simulink model "db6_4_Level_double"  (R2021a)
settings: Solver=VariableStepAuto  StartTime=0.0  StopTime=8  RelTol=1e-3
undefined symbols (not defined in the file): lambda2
libraries: dspsigops x9, dspquant2 x1
(part 2 of 3)

== system db6_4_Level_double/2nd_Level_Decomp/LoD_Even ==
  In_LoD_e : Inport  OutDataTypeStr=double  SampleTime=1/44100
  Add{,1..4} (5 alike) : Sum  AccumDataTypeStr=double  OutDataTypeStr=double
  Delay{,1..9} (10 alike) : Delay  DelayLength=1  SampleTime=1/44100
  LoD_0 : Constant  Value=-0.001077301  OutDataTypeStr=double  SampleTime=1/44100
  LoD_10 : Constant  Value=0.49462389  OutDataTypeStr=double  SampleTime=1/44100
  LoD_2 : Constant  Value=0.000553842  OutDataTypeStr=double  SampleTime=1/44100
  LoD_4 : Constant  Value=0.027522866  OutDataTypeStr=double  SampleTime=1/44100
  LoD_6 : Constant  Value=-0.129766868  OutDataTypeStr=double  SampleTime=1/44100
  LoD_8 : Constant  Value=0.315250352  OutDataTypeStr=double  SampleTime=1/44100
  Multiply{,1..5} (6 alike) : Product  OutDataTypeStr=double
  Rate Transition{,1..4} (5 alike) : RateTransition  OutPortSampleTime=1/44100
  Out_LoD_e : Outport  OutDataTypeStr=double  SampleTime=1/44100  VectorParamsAs1DForOutWhenUnconnected=off
  wires:
  Multiply3/1 -> Add3/1
  Add/1 -> Out_LoD_e/1
  Rate Transition3/1 -> Delay8/1, Multiply4/2
  Add3/1 -> Delay4/1
  In_LoD_e/1 -> Delay/1, Multiply/2
  Multiply2/1 -> Add2/1
  Multiply/1 -> Add/1
  Rate Transition1/1 -> Delay5/1, Multiply2/2
  Delay/1 -> Rate Transition/1
  Delay2/1 -> Add1/2
  Delay3/1 -> Add/2
  Delay7/1 -> Add3/2
  Add2/1 -> Delay2/1
  Add1/1 -> Delay3/1
  Rate Transition2/1 -> Delay6/1, Multiply3/2
  Delay1/1 -> Rate Transition1/1
  LoD_10/1 -> Multiply5/1
  Rate Transition/1 -> Delay1/1, Multiply1/2
  LoD_4/1 -> Multiply2/1
  Delay5/1 -> Rate Transition2/1
  LoD_0/1 -> Multiply/1
  LoD_2/1 -> Multiply1/1
  Delay8/1 -> Rate Transition4/1
  Rate Transition4/1 -> Multiply5/2
  Multiply4/1 -> Add4/1
  Delay4/1 -> Add2/2
  Delay9/1 -> Add4/2
  Multiply5/1 -> Delay9/1
  Delay6/1 -> Rate Transition3/1
  Add4/1 -> Delay7/1
  LoD_8/1 -> Multiply4/1
  LoD_6/1 -> Multiply3/1
  Multiply1/1 -> Add1/1

== system db6_4_Level_double/2nd_Level_Decomp/LoD_Odd ==
  In_LoD_o : Inport  OutDataTypeStr=double  SampleTime=1/44100
  Add{,1..4} (5 alike) : Sum  AccumDataTypeStr=double  OutDataTypeStr=double
  Delay{,1..9} (10 alike) : Delay  DelayLength=1  SampleTime=1/44100
  LoD_1 : Constant  Value=0.004777258  OutDataTypeStr=double  SampleTime=1/44100
  LoD_11 : Constant  Value=0.111540743  OutDataTypeStr=double  SampleTime=1/44100
  LoD_3 : Constant  Value=-0.031582039  OutDataTypeStr=double  SampleTime=1/44100
  LoD_5 : Constant  Value=0.097501606  OutDataTypeStr=double  SampleTime=1/44100
  LoD_7 : Constant  Value=-0.226264694  OutDataTypeStr=double  SampleTime=1/44100
  LoD_9 : Constant  Value=0.751133908  OutDataTypeStr=double  SampleTime=1/44100
  Multiply{,1..5} (6 alike) : Product  OutDataTypeStr=double
  Rate Transition{,1..4} (5 alike) : RateTransition  OutPortSampleTime=1/44100
  Out_LoD_o : Outport  OutDataTypeStr=double  SampleTime=1/44100  VectorParamsAs1DForOutWhenUnconnected=off
  wires:
  LoD_1/1 -> Multiply/1
  Delay/1 -> Rate Transition/1
  Multiply4/1 -> Add4/1
  Delay2/1 -> Add1/2
  Rate Transition2/1 -> Delay6/1, Multiply3/2
  LoD_7/1 -> Multiply3/1
  Delay7/1 -> Add3/2
  Add2/1 -> Delay2/1
  Add1/1 -> Delay3/1
  Delay3/1 -> Add/2
  Multiply5/1 -> Delay9/1
  Rate Transition4/1 -> Multiply5/2
  Delay8/1 -> Rate Transition4/1
  Delay9/1 -> Add4/2
  Delay5/1 -> Rate Transition2/1
  Add4/1 -> Delay7/1
  Rate Transition3/1 -> Delay8/1, Multiply4/2
  LoD_9/1 -> Multiply4/1
  LoD_5/1 -> Multiply2/1
  Rate Transition/1 -> Delay1/1, Multiply1/2
  LoD_3/1 -> Multiply1/1
  Multiply3/1 -> Add3/1
  Delay1/1 -> Rate Transition1/1
  Add3/1 -> Delay4/1
  Multiply/1 -> Add/1
  Multiply1/1 -> Add1/1
  In_LoD_o/1 -> Delay/1, Multiply/2
  Delay6/1 -> Rate Transition3/1
  Delay4/1 -> Add2/2
  Add/1 -> Out_LoD_o/1
  LoD_11/1 -> Multiply5/1
  Multiply2/1 -> Add2/1
  Rate Transition1/1 -> Delay5/1, Multiply2/2

== system db6_4_Level_double/2nd_Level_Recon/HiR_Even ==
  In_HiR_e : Inport  OutDataTypeStr=double  SampleTime=1/44100
  Add{,1..4} (5 alike) : Sum  AccumDataTypeStr=double  OutDataTypeStr=double
  Delay{,1..9} (10 alike) : Delay  DelayLength=1  SampleTime=1/44100
  HiR_0 : Constant  Value=-0.001077301  OutDataTypeStr=double  SampleTime=1/44100
  HiR_10 : Constant  Value=0.49462389  OutDataTypeStr=double  SampleTime=1/44100
  HiR_2 : Constant  Value=0.000553842  OutDataTypeStr=double  SampleTime=1/44100
  HiR_4 : Constant  Value=0.027522866  OutDataTypeStr=double  SampleTime=1/44100
  HiR_6 : Constant  Value=-0.129766868  OutDataTypeStr=double  SampleTime=1/44100
  HiR_8 : Constant  Value=0.315250352  OutDataTypeStr=double  SampleTime=1/44100
  Multiply{,1..5} (6 alike) : Product  OutDataTypeStr=double
  Rate Transition{,1..4} (5 alike) : RateTransition  OutPortSampleTime=1/44100
  Out_HiR_e : Outport  OutDataTypeStr=double  SampleTime=1/44100  VectorParamsAs1DForOutWhenUnconnected=off
  wires:
  Delay3/1 -> Add/2
  In_HiR_e/1 -> Delay/1, Multiply/2
  HiR_4/1 -> Multiply2/1
  Multiply/1 -> Add/1
  Add1/1 -> Delay3/1
  Multiply1/1 -> Add1/1
  Delay2/1 -> Add1/2
  Add/1 -> Out_HiR_e/1
  HiR_0/1 -> Multiply/1
  HiR_2/1 -> Multiply1/1
  Delay1/1 -> Rate Transition1/1
  Rate Transition/1 -> Delay1/1, Multiply1/2
  Rate Transition1/1 -> Delay4/1, Multiply2/2
  Delay/1 -> Rate Transition/1
  Delay4/1 -> Rate Transition2/1
  HiR_6/1 -> Multiply3/1
  Multiply2/1 -> Add2/1
  Add2/1 -> Delay2/1
  Delay5/1 -> Add2/2
  HiR_8/1 -> Multiply4/1
  Rate Transition2/1 -> Delay6/1, Multiply3/2
  Delay6/1 -> Rate Transition3/1
  Add3/1 -> Delay5/1
  Multiply3/1 -> Add3/1
  Delay7/1 -> Add3/2
  HiR_10/1 -> Multiply5/1
  Rate Transition3/1 -> Delay8/1, Multiply4/2
  Rate Transition4/1 -> Multiply5/2
  Delay8/1 -> Rate Transition4/1
  Multiply5/1 -> Delay9/1
  Add4/1 -> Delay7/1
  Multiply4/1 -> Add4/1
  Delay9/1 -> Add4/2

== system db6_4_Level_double/2nd_Level_Recon/HiR_Odd ==
  In_HiR_o : Inport  OutDataTypeStr=double  SampleTime=1/44100
  Add{,1..4} (5 alike) : Sum  AccumDataTypeStr=double  OutDataTypeStr=double
  Delay{,1..9} (10 alike) : Delay  DelayLength=1  SampleTime=1/44100
  HiR_1 : Constant  Value=-0.004777258  OutDataTypeStr=double  SampleTime=1/44100
  HiR_11 : Constant  Value=-0.111540743  OutDataTypeStr=double  SampleTime=1/44100
  HiR_3 : Constant  Value=0.031582039  OutDataTypeStr=double  SampleTime=1/44100
  HiR_5 : Constant  Value=-0.097501606  OutDataTypeStr=double  SampleTime=1/44100
  HiR_7 : Constant  Value=0.226264694  OutDataTypeStr=double  SampleTime=1/44100
  HiR_9 : Constant  Value=-0.751133908  OutDataTypeStr=double  SampleTime=1/44100
  Multiply{,1..5} (6 alike) : Product  OutDataTypeStr=double
  Rate Transition{,1..4} (5 alike) : RateTransition  OutPortSampleTime=1/44100
  Out_HiR_o : Outport  OutDataTypeStr=double  SampleTime=1/44100  VectorParamsAs1DForOutWhenUnconnected=off
  wires:
  HiR_7/1 -> Multiply3/1
  HiR_3/1 -> Multiply1/1
  Delay2/1 -> Add1/2
  Delay/1 -> Rate Transition/1
  Delay5/1 -> Add2/2
  HiR_5/1 -> Multiply2/1
  Delay4/1 -> Rate Transition2/1
  Delay3/1 -> Add/2
  Add2/1 -> Delay2/1
  Multiply/1 -> Add/1
  Multiply1/1 -> Add1/1
  Rate Transition2/1 -> Delay6/1, Multiply3/2
  HiR_1/1 -> Multiply/1
  Multiply5/1 -> Delay9/1
  Delay1/1 -> Rate Transition1/1
  Delay8/1 -> Rate Transition4/1
  Add1/1 -> Delay3/1
  Add4/1 -> Delay7/1
  Delay9/1 -> Add4/2
  Rate Transition1/1 -> Delay4/1, Multiply2/2
  Add3/1 -> Delay5/1
  Delay6/1 -> Rate Transition3/1
  Rate Transition/1 -> Delay1/1, Multiply1/2
  HiR_9/1 -> Multiply4/1
  Multiply4/1 -> Add4/1
  Delay7/1 -> Add3/2
  Multiply3/1 -> Add3/1
  Multiply2/1 -> Add2/1
  HiR_11/1 -> Multiply5/1
  Rate Transition3/1 -> Delay8/1, Multiply4/2
  Add/1 -> Out_HiR_o/1
  In_HiR_o/1 -> Delay/1, Multiply/2
  Rate Transition4/1 -> Multiply5/2

== system db6_4_Level_double/2nd_Level_Recon/LoR_Even ==
  In_LoR_e : Inport  OutDataTypeStr=double  SampleTime=1/44100
  Add{,1..4} (5 alike) : Sum  AccumDataTypeStr=double  OutDataTypeStr=double
  Delay{,1..9} (10 alike) : Delay  DelayLength=1  SampleTime=1/44100
  LoR_0 : Constant  Value=0.111540743  OutDataTypeStr=double  SampleTime=1/44100
  LoR_10 : Constant  Value=0.004777258  OutDataTypeStr=double  SampleTime=1/44100
  LoR_2 : Constant  Value=0.751133908  OutDataTypeStr=double  SampleTime=1/44100
  LoR_4 : Constant  Value=-0.226264694  OutDataTypeStr=double  SampleTime=1/44100
  LoR_6 : Constant  Value=0.097501606  OutDataTypeStr=double  SampleTime=1/44100
  LoR_8 : Constant  Value=-0.031582039  OutDataTypeStr=double  SampleTime=1/44100
  Multiply{,1..5} (6 alike) : Product  OutDataTypeStr=double
  Rate Transition{,1..4} (5 alike) : RateTransition  OutPortSampleTime=1/44100
  Out_LoR_e : Outport  OutDataTypeStr=double  SampleTime=1/44100  VectorParamsAs1DForOutWhenUnconnected=off
  wires:
  Multiply5/1 -> Delay9/1
  LoR_6/1 -> Multiply3/1
  Rate Transition2/1 -> Delay6/1, Multiply3/2
  Multiply1/1 -> Add1/1
  Multiply/1 -> Add/1
  LoR_8/1 -> Multiply4/1
  Rate Transition3/1 -> Delay8/1, Multiply4/2
  Add2/1 -> Delay2/1
  Delay5/1 -> Add2/2
  Multiply2/1 -> Add2/1
  Delay3/1 -> Add/2
  Delay4/1 -> Rate Transition2/1
  Delay2/1 -> Add1/2
  Delay/1 -> Rate Transition/1
  In_LoR_e/1 -> Delay/1, Multiply/2
  Rate Transition/1 -> Delay1/1, Multiply1/2
  Add1/1 -> Delay3/1
  Add3/1 -> Delay5/1
  Delay8/1 -> Rate Transition4/1
  Delay1/1 -> Rate Transition1/1
  Delay6/1 -> Rate Transition3/1
  Rate Transition1/1 -> Delay4/1, Multiply2/2
  Delay9/1 -> Add4/2
  LoR_4/1 -> Multiply2/1
  Add4/1 -> Delay7/1
  LoR_0/1 -> Multiply/1
  Rate Transition4/1 -> Multiply5/2
  Multiply3/1 -> Add3/1
  Multiply4/1 -> Add4/1
  LoR_2/1 -> Multiply1/1
  Delay7/1 -> Add3/2
  LoR_10/1 -> Multiply5/1
  Add/1 -> Out_LoR_e/1

== system db6_4_Level_double/2nd_Level_Recon/LoR_Odd ==
  In_LoR_o : Inport  OutDataTypeStr=double  SampleTime=1/44100
  Add{,1..4} (5 alike) : Sum  AccumDataTypeStr=double  OutDataTypeStr=double
  Delay{,1..9} (10 alike) : Delay  DelayLength=1  SampleTime=1/44100
  LoR_1 : Constant  Value=0.49462389  OutDataTypeStr=double  SampleTime=1/44100
  LoR_11 : Constant  Value=-0.001077301  OutDataTypeStr=double  SampleTime=1/44100
  LoR_3 : Constant  Value=0.315250352  OutDataTypeStr=double  SampleTime=1/44100
  LoR_5 : Constant  Value=-0.129766868  OutDataTypeStr=double  SampleTime=1/44100
  LoR_7 : Constant  Value=0.027522866  OutDataTypeStr=double  SampleTime=1/44100
  LoR_9 : Constant  Value=0.000553842  OutDataTypeStr=double  SampleTime=1/44100
  Multiply{,1..5} (6 alike) : Product  OutDataTypeStr=double
  Rate Transition{,1..4} (5 alike) : RateTransition  OutPortSampleTime=1/44100
  Out_LoR_o : Outport  OutDataTypeStr=double  SampleTime=1/44100  VectorParamsAs1DForOutWhenUnconnected=off
  wires:
  Rate Transition2/1 -> Delay6/1, Multiply3/2
  Delay3/1 -> Add/2
  Add2/1 -> Delay2/1
  Delay4/1 -> Rate Transition2/1
  Delay/1 -> Rate Transition/1
  Delay5/1 -> Add2/2
  Delay2/1 -> Add1/2
  LoR_5/1 -> Multiply2/1
  LoR_7/1 -> Multiply3/1
  LoR_1/1 -> Multiply/1
  Multiply5/1 -> Delay9/1
  Multiply4/1 -> Add4/1
  LoR_11/1 -> Multiply5/1
  Rate Transition/1 -> Delay1/1, Multiply1/2
  Multiply/1 -> Add/1
  Delay6/1 -> Rate Transition3/1
  Add3/1 -> Delay5/1
  Rate Transition1/1 -> Delay4/1, Multiply2/2
  Add4/1 -> Delay7/1
  Delay9/1 -> Add4/2
  Add1/1 -> Delay3/1
  Delay8/1 -> Rate Transition4/1
  In_LoR_o/1 -> Delay/1, Multiply/2
  Add/1 -> Out_LoR_o/1
  Rate Transition3/1 -> Delay8/1, Multiply4/2
  Multiply1/1 -> Add1/1
  Rate Transition4/1 -> Multiply5/2
  LoR_9/1 -> Multiply4/1
  Delay1/1 -> Rate Transition1/1
  Delay7/1 -> Add3/2
  LoR_3/1 -> Multiply1/1
  Multiply3/1 -> Add3/1
  Multiply2/1 -> Add2/1

== system db6_4_Level_double/3rd_Level_Decomp/HiD_Even ==
  In_HiD_e : Inport  OutDataTypeStr=double  SampleTime=1/44100
  Add{,1..4} (5 alike) : Sum  AccumDataTypeStr=double  OutDataTypeStr=double
  Delay{,1..9} (10 alike) : Delay  DelayLength=1  SampleTime=1/44100
  HiD_0 : Constant  Value=-0.111540743  OutDataTypeStr=double  SampleTime=1/44100
  HiD_10 : Constant  Value=-0.004777258  OutDataTypeStr=double  SampleTime=1/44100
  HiD_2 : Constant  Value=-0.751133908  OutDataTypeStr=double  SampleTime=1/44100
  HiD_4 : Constant  Value=0.226264694  OutDataTypeStr=double  SampleTime=1/44100
  HiD_6 : Constant  Value=-0.097501606  OutDataTypeStr=double  SampleTime=1/44100
  HiD_8 : Constant  Value=0.031582039  OutDataTypeStr=double  SampleTime=1/44100
  Multiply{,1..5} (6 alike) : Product  OutDataTypeStr=double
  Rate Transition{,1..4} (5 alike) : RateTransition  OutPortSampleTime=1/44100
  Out_HiD_e : Outport  OutDataTypeStr=double  SampleTime=1/44100  VectorParamsAs1DForOutWhenUnconnected=off
  wires:
  Delay1/1 -> Rate Transition1/1
  Delay3/1 -> Add/2
  HiD_2/1 -> Multiply1/1
  Rate Transition2/1 -> Delay6/1, Multiply3/2
  Add/1 -> Out_HiD_e/1
  Delay4/1 -> Add2/2
  Delay5/1 -> Rate Transition2/1
  Rate Transition1/1 -> Delay5/1, Multiply2/2
  HiD_0/1 -> Multiply/1
  Multiply2/1 -> Add2/1
  Add2/1 -> Delay2/1
  HiD_6/1 -> Multiply3/1
  Multiply/1 -> Add/1
  In_HiD_e/1 -> Delay/1, Multiply/2
  Multiply1/1 -> Add1/1
  Rate Transition/1 -> Delay1/1, Multiply1/2
  Add1/1 -> Delay3/1
  HiD_4/1 -> Multiply2/1
  Delay/1 -> Rate Transition/1
  Delay2/1 -> Add1/2
  HiD_8/1 -> Multiply4/1
  Delay6/1 -> Rate Transition3/1
  Multiply3/1 -> Add3/1
  Add3/1 -> Delay4/1
  Delay7/1 -> Add3/2
  HiD_10/1 -> Multiply5/1
  Rate Transition4/1 -> Multiply5/2
  Multiply5/1 -> Delay9/1
  Rate Transition3/1 -> Delay8/1, Multiply4/2
  Delay8/1 -> Rate Transition4/1
  Add4/1 -> Delay7/1
  Multiply4/1 -> Add4/1
  Delay9/1 -> Add4/2

== system db6_4_Level_double/3rd_Level_Decomp/HiD_Odd ==
  In_HiD_o : Inport  OutDataTypeStr=double  SampleTime=1/44100
  Add{,1..4} (5 alike) : Sum  AccumDataTypeStr=double  OutDataTypeStr=double
  Delay{,1..9} (10 alike) : Delay  DelayLength=1  SampleTime=1/44100
  HiD_1 : Constant  Value=0.49462389  OutDataTypeStr=double  SampleTime=1/44100
  HiD_11 : Constant  Value=-0.001077301  OutDataTypeStr=double  SampleTime=1/44100
  HiD_3 : Constant  Value=0.315250352  OutDataTypeStr=double  SampleTime=1/44100
  HiD_5 : Constant  Value=-0.129766868  OutDataTypeStr=double  SampleTime=1/44100
  HiD_7 : Constant  Value=0.027522866  OutDataTypeStr=double  SampleTime=1/44100
  HiD_9 : Constant  Value=0.000553842  OutDataTypeStr=double  SampleTime=1/44100
  Multiply{,1..5} (6 alike) : Product  OutDataTypeStr=double
  Rate Transition{,1..4} (5 alike) : RateTransition  OutPortSampleTime=1/44100
  Out_HiD_o : Outport  OutDataTypeStr=double  SampleTime=1/44100  VectorParamsAs1DForOutWhenUnconnected=off
  wires:
  HiD_7/1 -> Multiply3/1
  HiD_3/1 -> Multiply1/1
  HiD_5/1 -> Multiply2/1
  Add/1 -> Out_HiD_o/1
  HiD_9/1 -> Multiply4/1
  Add3/1 -> Delay4/1
  Multiply3/1 -> Add3/1
  Multiply2/1 -> Add2/1
  In_HiD_o/1 -> Delay/1, Multiply/2
  HiD_11/1 -> Multiply5/1
  Multiply1/1 -> Add1/1
  Delay4/1 -> Add2/2
  Delay6/1 -> Rate Transition3/1
  Rate Transition3/1 -> Delay8/1, Multiply4/2
  Delay9/1 -> Add4/2
  Add4/1 -> Delay7/1
  Delay8/1 -> Rate Transition4/1
  Delay5/1 -> Rate Transition2/1
  Rate Transition4/1 -> Multiply5/2
  HiD_1/1 -> Multiply/1
  Delay1/1 -> Rate Transition1/1
  Add1/1 -> Delay3/1
  Add2/1 -> Delay2/1
  Multiply5/1 -> Delay9/1
  Rate Transition2/1 -> Delay6/1, Multiply3/2
  Delay7/1 -> Add3/2
  Rate Transition/1 -> Delay1/1, Multiply1/2
  Rate Transition1/1 -> Delay5/1, Multiply2/2
  Multiply/1 -> Add/1
  Delay/1 -> Rate Transition/1
  Multiply4/1 -> Add4/1
  Delay3/1 -> Add/2
  Delay2/1 -> Add1/2

== system db6_4_Level_double/3rd_Level_Decomp/LoD_Even ==
  In_LoD_e : Inport  OutDataTypeStr=double  SampleTime=1/44100
  Add{,1..4} (5 alike) : Sum  AccumDataTypeStr=double  OutDataTypeStr=double
  Delay{,1..9} (10 alike) : Delay  DelayLength=1  SampleTime=1/44100
  LoD_0 : Constant  Value=-0.001077301  OutDataTypeStr=double  SampleTime=1/44100
  LoD_10 : Constant  Value=0.49462389  OutDataTypeStr=double  SampleTime=1/44100
  LoD_2 : Constant  Value=0.000553842  OutDataTypeStr=double  SampleTime=1/44100
  LoD_4 : Constant  Value=0.027522866  OutDataTypeStr=double  SampleTime=1/44100
  LoD_6 : Constant  Value=-0.129766868  OutDataTypeStr=double  SampleTime=1/44100
  LoD_8 : Constant  Value=0.315250352  OutDataTypeStr=double  SampleTime=1/44100
  Multiply{,1..5} (6 alike) : Product  OutDataTypeStr=double
  Rate Transition{,1..4} (5 alike) : RateTransition  OutPortSampleTime=1/44100
  Out_LoD_e : Outport  OutDataTypeStr=double  SampleTime=1/44100  VectorParamsAs1DForOutWhenUnconnected=off
  wires:
  Multiply3/1 -> Add3/1
  Add/1 -> Out_LoD_e/1
  Rate Transition3/1 -> Delay8/1, Multiply4/2
  Add3/1 -> Delay4/1
  In_LoD_e/1 -> Delay/1, Multiply/2
  Multiply2/1 -> Add2/1
  Multiply/1 -> Add/1
  Rate Transition1/1 -> Delay5/1, Multiply2/2
  Delay/1 -> Rate Transition/1
  Delay2/1 -> Add1/2
  Delay3/1 -> Add/2
  Delay7/1 -> Add3/2
  Add2/1 -> Delay2/1
  Add1/1 -> Delay3/1
  Rate Transition2/1 -> Delay6/1, Multiply3/2
  Delay1/1 -> Rate Transition1/1
  LoD_10/1 -> Multiply5/1
  Rate Transition/1 -> Delay1/1, Multiply1/2
  LoD_4/1 -> Multiply2/1
  Delay5/1 -> Rate Transition2/1
  LoD_0/1 -> Multiply/1
  LoD_2/1 -> Multiply1/1
  Delay8/1 -> Rate Transition4/1
  Rate Transition4/1 -> Multiply5/2
  Multiply4/1 -> Add4/1
  Delay4/1 -> Add2/2
  Delay9/1 -> Add4/2
  Multiply5/1 -> Delay9/1
  Delay6/1 -> Rate Transition3/1
  Add4/1 -> Delay7/1
  LoD_8/1 -> Multiply4/1
  LoD_6/1 -> Multiply3/1
  Multiply1/1 -> Add1/1

== system db6_4_Level_double/3rd_Level_Decomp/LoD_Odd ==
  In_LoD_o : Inport  OutDataTypeStr=double  SampleTime=1/44100
  Add{,1..4} (5 alike) : Sum  AccumDataTypeStr=double  OutDataTypeStr=double
  Delay{,1..9} (10 alike) : Delay  DelayLength=1  SampleTime=1/44100
  LoD_1 : Constant  Value=0.004777258  OutDataTypeStr=double  SampleTime=1/44100
  LoD_11 : Constant  Value=0.111540743  OutDataTypeStr=double  SampleTime=1/44100
  LoD_3 : Constant  Value=-0.031582039  OutDataTypeStr=double  SampleTime=1/44100
  LoD_5 : Constant  Value=0.097501606  OutDataTypeStr=double  SampleTime=1/44100
  LoD_7 : Constant  Value=-0.226264694  OutDataTypeStr=double  SampleTime=1/44100
  LoD_9 : Constant  Value=0.751133908  OutDataTypeStr=double  SampleTime=1/44100
  Multiply{,1..5} (6 alike) : Product  OutDataTypeStr=double
  Rate Transition{,1..4} (5 alike) : RateTransition  OutPortSampleTime=1/44100
  Out_LoD_o : Outport  OutDataTypeStr=double  SampleTime=1/44100  VectorParamsAs1DForOutWhenUnconnected=off
  wires:
  LoD_1/1 -> Multiply/1
  Delay/1 -> Rate Transition/1
  Multiply4/1 -> Add4/1
  Delay2/1 -> Add1/2
  Rate Transition2/1 -> Delay6/1, Multiply3/2
  LoD_7/1 -> Multiply3/1
  Delay7/1 -> Add3/2
  Add2/1 -> Delay2/1
  Add1/1 -> Delay3/1
  Delay3/1 -> Add/2
  Multiply5/1 -> Delay9/1
  Rate Transition4/1 -> Multiply5/2
  Delay8/1 -> Rate Transition4/1
  Delay9/1 -> Add4/2
  Delay5/1 -> Rate Transition2/1
  Add4/1 -> Delay7/1
  Rate Transition3/1 -> Delay8/1, Multiply4/2
  LoD_9/1 -> Multiply4/1
  LoD_5/1 -> Multiply2/1
  Rate Transition/1 -> Delay1/1, Multiply1/2
  LoD_3/1 -> Multiply1/1
  Multiply3/1 -> Add3/1
  Delay1/1 -> Rate Transition1/1
  Add3/1 -> Delay4/1
  Multiply/1 -> Add/1
  Multiply1/1 -> Add1/1
  In_LoD_o/1 -> Delay/1, Multiply/2
  Delay6/1 -> Rate Transition3/1
  Delay4/1 -> Add2/2
  Add/1 -> Out_LoD_o/1
  LoD_11/1 -> Multiply5/1
  Multiply2/1 -> Add2/1
  Rate Transition1/1 -> Delay5/1, Multiply2/2

== system db6_4_Level_double/3rd_Level_Recon/HiR_Even ==
  In_HiR_e : Inport  OutDataTypeStr=double  SampleTime=1/44100
  Add{,1..4} (5 alike) : Sum  AccumDataTypeStr=double  OutDataTypeStr=double
  Delay{,1..9} (10 alike) : Delay  DelayLength=1  SampleTime=1/44100
  HiR_0 : Constant  Value=-0.001077301  OutDataTypeStr=double  SampleTime=1/44100
  HiR_10 : Constant  Value=0.49462389  OutDataTypeStr=double  SampleTime=1/44100
  HiR_2 : Constant  Value=0.000553842  OutDataTypeStr=double  SampleTime=1/44100
  HiR_4 : Constant  Value=0.027522866  OutDataTypeStr=double  SampleTime=1/44100
  HiR_6 : Constant  Value=-0.129766868  OutDataTypeStr=double  SampleTime=1/44100
  HiR_8 : Constant  Value=0.315250352  OutDataTypeStr=double  SampleTime=1/44100
  Multiply{,1..5} (6 alike) : Product  OutDataTypeStr=double
  Rate Transition{,1..4} (5 alike) : RateTransition  OutPortSampleTime=1/44100
  Out_HiR_e : Outport  OutDataTypeStr=double  SampleTime=1/44100  VectorParamsAs1DForOutWhenUnconnected=off
  wires:
  Delay3/1 -> Add/2
  In_HiR_e/1 -> Delay/1, Multiply/2
  HiR_4/1 -> Multiply2/1
  Multiply/1 -> Add/1
  Add1/1 -> Delay3/1
  Multiply1/1 -> Add1/1
  Delay2/1 -> Add1/2
  Add/1 -> Out_HiR_e/1
  HiR_0/1 -> Multiply/1
  HiR_2/1 -> Multiply1/1
  Delay1/1 -> Rate Transition1/1
  Rate Transition/1 -> Delay1/1, Multiply1/2
  Rate Transition1/1 -> Delay4/1, Multiply2/2
  Delay/1 -> Rate Transition/1
  Delay4/1 -> Rate Transition2/1
  HiR_6/1 -> Multiply3/1
  Multiply2/1 -> Add2/1
  Add2/1 -> Delay2/1
  Delay5/1 -> Add2/2
  HiR_8/1 -> Multiply4/1
  Rate Transition2/1 -> Delay6/1, Multiply3/2
  Delay6/1 -> Rate Transition3/1
  Add3/1 -> Delay5/1
  Multiply3/1 -> Add3/1
  Delay7/1 -> Add3/2
  HiR_10/1 -> Multiply5/1
  Rate Transition3/1 -> Delay8/1, Multiply4/2
  Rate Transition4/1 -> Multiply5/2
  Delay8/1 -> Rate Transition4/1
  Multiply5/1 -> Delay9/1
  Add4/1 -> Delay7/1
  Multiply4/1 -> Add4/1
  Delay9/1 -> Add4/2

== system db6_4_Level_double/3rd_Level_Recon/HiR_Odd ==
  In_HiR_o : Inport  OutDataTypeStr=double  SampleTime=1/44100
  Add{,1..4} (5 alike) : Sum  AccumDataTypeStr=double  OutDataTypeStr=double
  Delay{,1..9} (10 alike) : Delay  DelayLength=1  SampleTime=1/44100
  HiR_1 : Constant  Value=-0.004777258  OutDataTypeStr=double  SampleTime=1/44100
  HiR_11 : Constant  Value=-0.111540743  OutDataTypeStr=double  SampleTime=1/44100
  HiR_3 : Constant  Value=0.031582039  OutDataTypeStr=double  SampleTime=1/44100
  HiR_5 : Constant  Value=-0.097501606  OutDataTypeStr=double  SampleTime=1/44100
  HiR_7 : Constant  Value=0.226264694  OutDataTypeStr=double  SampleTime=1/44100
  HiR_9 : Constant  Value=-0.751133908  OutDataTypeStr=double  SampleTime=1/44100
  Multiply{,1..5} (6 alike) : Product  OutDataTypeStr=double
  Rate Transition{,1..4} (5 alike) : RateTransition  OutPortSampleTime=1/44100
  Out_HiR_o : Outport  OutDataTypeStr=double  SampleTime=1/44100  VectorParamsAs1DForOutWhenUnconnected=off
  wires:
  HiR_7/1 -> Multiply3/1
  HiR_3/1 -> Multiply1/1
  Delay2/1 -> Add1/2
  Delay/1 -> Rate Transition/1
  Delay5/1 -> Add2/2
  HiR_5/1 -> Multiply2/1
  Delay4/1 -> Rate Transition2/1
  Delay3/1 -> Add/2
  Add2/1 -> Delay2/1
  Multiply/1 -> Add/1
  Multiply1/1 -> Add1/1
  Rate Transition2/1 -> Delay6/1, Multiply3/2
  HiR_1/1 -> Multiply/1
  Multiply5/1 -> Delay9/1
  Delay1/1 -> Rate Transition1/1
  Delay8/1 -> Rate Transition4/1
  Add1/1 -> Delay3/1
  Add4/1 -> Delay7/1
  Delay9/1 -> Add4/2
  Rate Transition1/1 -> Delay4/1, Multiply2/2
  Add3/1 -> Delay5/1
  Delay6/1 -> Rate Transition3/1
  Rate Transition/1 -> Delay1/1, Multiply1/2
  HiR_9/1 -> Multiply4/1
  Multiply4/1 -> Add4/1
  Delay7/1 -> Add3/2
  Multiply3/1 -> Add3/1
  Multiply2/1 -> Add2/1
  HiR_11/1 -> Multiply5/1
  Rate Transition3/1 -> Delay8/1, Multiply4/2
  Add/1 -> Out_HiR_o/1
  In_HiR_o/1 -> Delay/1, Multiply/2
  Rate Transition4/1 -> Multiply5/2

== system db6_4_Level_double/3rd_Level_Recon/LoR_Even ==
  In_LoR_e : Inport  OutDataTypeStr=double  SampleTime=1/44100
  Add{,1..4} (5 alike) : Sum  AccumDataTypeStr=double  OutDataTypeStr=double
  Delay{,1..9} (10 alike) : Delay  DelayLength=1  SampleTime=1/44100
  LoR_0 : Constant  Value=0.111540743  OutDataTypeStr=double  SampleTime=1/44100
  LoR_10 : Constant  Value=0.004777258  OutDataTypeStr=double  SampleTime=1/44100
  LoR_2 : Constant  Value=0.751133908  OutDataTypeStr=double  SampleTime=1/44100
  LoR_4 : Constant  Value=-0.226264694  OutDataTypeStr=double  SampleTime=1/44100
  LoR_6 : Constant  Value=0.097501606  OutDataTypeStr=double  SampleTime=1/44100
  LoR_8 : Constant  Value=-0.031582039  OutDataTypeStr=double  SampleTime=1/44100
  Multiply{,1..5} (6 alike) : Product  OutDataTypeStr=double
  Rate Transition{,1..4} (5 alike) : RateTransition  OutPortSampleTime=1/44100
  Out_LoR_e : Outport  OutDataTypeStr=double  SampleTime=1/44100  VectorParamsAs1DForOutWhenUnconnected=off
  wires:
  Multiply5/1 -> Delay9/1
  LoR_6/1 -> Multiply3/1
  Rate Transition2/1 -> Delay6/1, Multiply3/2
  Multiply1/1 -> Add1/1
  Multiply/1 -> Add/1
  LoR_8/1 -> Multiply4/1
  Rate Transition3/1 -> Delay8/1, Multiply4/2
  Add2/1 -> Delay2/1
  Delay5/1 -> Add2/2
  Multiply2/1 -> Add2/1
  Delay3/1 -> Add/2
  Delay4/1 -> Rate Transition2/1
  Delay2/1 -> Add1/2
  Delay/1 -> Rate Transition/1
  In_LoR_e/1 -> Delay/1, Multiply/2
  Rate Transition/1 -> Delay1/1, Multiply1/2
  Add1/1 -> Delay3/1
  Add3/1 -> Delay5/1
  Delay8/1 -> Rate Transition4/1
  Delay1/1 -> Rate Transition1/1
  Delay6/1 -> Rate Transition3/1
  Rate Transition1/1 -> Delay4/1, Multiply2/2
  Delay9/1 -> Add4/2
  LoR_4/1 -> Multiply2/1
  Add4/1 -> Delay7/1
  LoR_0/1 -> Multiply/1
  Rate Transition4/1 -> Multiply5/2
  Multiply3/1 -> Add3/1
  Multiply4/1 -> Add4/1
  LoR_2/1 -> Multiply1/1
  Delay7/1 -> Add3/2
  LoR_10/1 -> Multiply5/1
  Add/1 -> Out_LoR_e/1

== system db6_4_Level_double/3rd_Level_Recon/LoR_Odd ==
  In_LoR_o : Inport  OutDataTypeStr=double  SampleTime=1/44100
  Add{,1..4} (5 alike) : Sum  AccumDataTypeStr=double  OutDataTypeStr=double
  Delay{,1..9} (10 alike) : Delay  DelayLength=1  SampleTime=1/44100
  LoR_1 : Constant  Value=0.49462389  OutDataTypeStr=double  SampleTime=1/44100
  LoR_11 : Constant  Value=-0.001077301  OutDataTypeStr=double  SampleTime=1/44100
  LoR_3 : Constant  Value=0.315250352  OutDataTypeStr=double  SampleTime=1/44100
  LoR_5 : Constant  Value=-0.129766868  OutDataTypeStr=double  SampleTime=1/44100
  LoR_7 : Constant  Value=0.027522866  OutDataTypeStr=double  SampleTime=1/44100
  LoR_9 : Constant  Value=0.000553842  OutDataTypeStr=double  SampleTime=1/44100
  Multiply{,1..5} (6 alike) : Product  OutDataTypeStr=double
  Rate Transition{,1..4} (5 alike) : RateTransition  OutPortSampleTime=1/44100
  Out_LoR_o : Outport  OutDataTypeStr=double  SampleTime=1/44100  VectorParamsAs1DForOutWhenUnconnected=off
  wires:
  Rate Transition2/1 -> Delay6/1, Multiply3/2
  Delay3/1 -> Add/2
  Add2/1 -> Delay2/1
  Delay4/1 -> Rate Transition2/1
  Delay/1 -> Rate Transition/1
  Delay5/1 -> Add2/2
  Delay2/1 -> Add1/2
  LoR_5/1 -> Multiply2/1
  LoR_7/1 -> Multiply3/1
  LoR_1/1 -> Multiply/1
  Multiply5/1 -> Delay9/1
  Multiply4/1 -> Add4/1
  LoR_11/1 -> Multiply5/1
  Rate Transition/1 -> Delay1/1, Multiply1/2
  Multiply/1 -> Add/1
  Delay6/1 -> Rate Transition3/1
  Add3/1 -> Delay5/1
  Rate Transition1/1 -> Delay4/1, Multiply2/2
  Add4/1 -> Delay7/1
  Delay9/1 -> Add4/2
  Add1/1 -> Delay3/1
  Delay8/1 -> Rate Transition4/1
  In_LoR_o/1 -> Delay/1, Multiply/2
  Add/1 -> Out_LoR_o/1
  Rate Transition3/1 -> Delay8/1, Multiply4/2
  Multiply1/1 -> Add1/1
  Rate Transition4/1 -> Multiply5/2
  LoR_9/1 -> Multiply4/1
  Delay1/1 -> Rate Transition1/1
  Delay7/1 -> Add3/2
  LoR_3/1 -> Multiply1/1
  Multiply3/1 -> Add3/1
  Multiply2/1 -> Add2/1

== system db6_4_Level_double/4th_Level_Decomp/HiD_Even ==
  In_HiD_e : Inport  OutDataTypeStr=double  SampleTime=1/44100
  Add{,1..4} (5 alike) : Sum  AccumDataTypeStr=double  OutDataTypeStr=double
  Delay{,1..9} (10 alike) : Delay  DelayLength=1  SampleTime=1/44100
  HiD_0 : Constant  Value=-0.111540743  OutDataTypeStr=double  SampleTime=1/44100
  HiD_10 : Constant  Value=-0.004777258  OutDataTypeStr=double  SampleTime=1/44100
  HiD_2 : Constant  Value=-0.751133908  OutDataTypeStr=double  SampleTime=1/44100
  HiD_4 : Constant  Value=0.226264694  OutDataTypeStr=double  SampleTime=1/44100
  HiD_6 : Constant  Value=-0.097501606  OutDataTypeStr=double  SampleTime=1/44100
  HiD_8 : Constant  Value=0.031582039  OutDataTypeStr=double  SampleTime=1/44100
  Multiply{,1..5} (6 alike) : Product  OutDataTypeStr=double
  Rate Transition{,1..4} (5 alike) : RateTransition  OutPortSampleTime=1/44100
  Out_HiD_e : Outport  OutDataTypeStr=double  SampleTime=1/44100  VectorParamsAs1DForOutWhenUnconnected=off
  wires:
  Delay1/1 -> Rate Transition1/1
  Delay3/1 -> Add/2
  HiD_2/1 -> Multiply1/1
  Rate Transition2/1 -> Delay6/1, Multiply3/2
  Add/1 -> Out_HiD_e/1
  Delay4/1 -> Add2/2
  Delay5/1 -> Rate Transition2/1
  Rate Transition1/1 -> Delay5/1, Multiply2/2
  HiD_0/1 -> Multiply/1
  Multiply2/1 -> Add2/1
  Add2/1 -> Delay2/1
  HiD_6/1 -> Multiply3/1
  Multiply/1 -> Add/1
  In_HiD_e/1 -> Delay/1, Multiply/2
  Multiply1/1 -> Add1/1
  Rate Transition/1 -> Delay1/1, Multiply1/2
  Add1/1 -> Delay3/1
  HiD_4/1 -> Multiply2/1
  Delay/1 -> Rate Transition/1
  Delay2/1 -> Add1/2
  HiD_8/1 -> Multiply4/1
  Delay6/1 -> Rate Transition3/1
  Multiply3/1 -> Add3/1
  Add3/1 -> Delay4/1
  Delay7/1 -> Add3/2
  HiD_10/1 -> Multiply5/1
  Rate Transition4/1 -> Multiply5/2
  Multiply5/1 -> Delay9/1
  Rate Transition3/1 -> Delay8/1, Multiply4/2
  Delay8/1 -> Rate Transition4/1
  Add4/1 -> Delay7/1
  Multiply4/1 -> Add4/1
  Delay9/1 -> Add4/2

== system db6_4_Level_double/4th_Level_Decomp/HiD_Odd ==
  In_HiD_o : Inport  OutDataTypeStr=double  SampleTime=1/44100
  Add{,1..4} (5 alike) : Sum  AccumDataTypeStr=double  OutDataTypeStr=double
  Delay{,1..9} (10 alike) : Delay  DelayLength=1  SampleTime=1/44100
  HiD_1 : Constant  Value=0.49462389  OutDataTypeStr=double  SampleTime=1/44100
  HiD_11 : Constant  Value=-0.001077301  OutDataTypeStr=double  SampleTime=1/44100
  HiD_3 : Constant  Value=0.315250352  OutDataTypeStr=double  SampleTime=1/44100
  HiD_5 : Constant  Value=-0.129766868  OutDataTypeStr=double  SampleTime=1/44100
  HiD_7 : Constant  Value=0.027522866  OutDataTypeStr=double  SampleTime=1/44100
  HiD_9 : Constant  Value=0.000553842  OutDataTypeStr=double  SampleTime=1/44100
  Multiply{,1..5} (6 alike) : Product  OutDataTypeStr=double
  Rate Transition{,1..4} (5 alike) : RateTransition  OutPortSampleTime=1/44100
  Out_HiD_o : Outport  OutDataTypeStr=double  SampleTime=1/44100  VectorParamsAs1DForOutWhenUnconnected=off
  wires:
  HiD_7/1 -> Multiply3/1
  HiD_3/1 -> Multiply1/1
  HiD_5/1 -> Multiply2/1
  Add/1 -> Out_HiD_o/1
  HiD_9/1 -> Multiply4/1
  Add3/1 -> Delay4/1
  Multiply3/1 -> Add3/1
  Multiply2/1 -> Add2/1
  In_HiD_o/1 -> Delay/1, Multiply/2
  HiD_11/1 -> Multiply5/1
  Multiply1/1 -> Add1/1
  Delay4/1 -> Add2/2
  Delay6/1 -> Rate Transition3/1
  Rate Transition3/1 -> Delay8/1, Multiply4/2
  Delay9/1 -> Add4/2
  Add4/1 -> Delay7/1
  Delay8/1 -> Rate Transition4/1
  Delay5/1 -> Rate Transition2/1
  Rate Transition4/1 -> Multiply5/2
  HiD_1/1 -> Multiply/1
  Delay1/1 -> Rate Transition1/1
  Add1/1 -> Delay3/1
  Add2/1 -> Delay2/1
  Multiply5/1 -> Delay9/1
  Rate Transition2/1 -> Delay6/1, Multiply3/2
  Delay7/1 -> Add3/2
  Rate Transition/1 -> Delay1/1, Multiply1/2
  Rate Transition1/1 -> Delay5/1, Multiply2/2
  Multiply/1 -> Add/1
  Delay/1 -> Rate Transition/1
  Multiply4/1 -> Add4/1
  Delay3/1 -> Add/2
  Delay2/1 -> Add1/2

== system db6_4_Level_double/4th_Level_Decomp/LoD_Even ==
  In_LoD_e : Inport  OutDataTypeStr=double  SampleTime=1/44100
  Add{,1..4} (5 alike) : Sum  AccumDataTypeStr=double  OutDataTypeStr=double
  Delay{,1..9} (10 alike) : Delay  DelayLength=1  SampleTime=1/44100
  LoD_0 : Constant  Value=-0.001077301  OutDataTypeStr=double  SampleTime=1/44100
  LoD_10 : Constant  Value=0.49462389  OutDataTypeStr=double  SampleTime=1/44100
  LoD_2 : Constant  Value=0.000553842  OutDataTypeStr=double  SampleTime=1/44100
  LoD_4 : Constant  Value=0.027522866  OutDataTypeStr=double  SampleTime=1/44100
  LoD_6 : Constant  Value=-0.129766868  OutDataTypeStr=double  SampleTime=1/44100
  LoD_8 : Constant  Value=0.315250352  OutDataTypeStr=double  SampleTime=1/44100
  Multiply{,1..5} (6 alike) : Product  OutDataTypeStr=double
  Rate Transition{,1..4} (5 alike) : RateTransition  OutPortSampleTime=1/44100
  Out_LoD_e : Outport  OutDataTypeStr=double  SampleTime=1/44100  VectorParamsAs1DForOutWhenUnconnected=off
  wires:
  Multiply3/1 -> Add3/1
  Add/1 -> Out_LoD_e/1
  Rate Transition3/1 -> Delay8/1, Multiply4/2
  Add3/1 -> Delay4/1
  In_LoD_e/1 -> Delay/1, Multiply/2
  Multiply2/1 -> Add2/1
  Multiply/1 -> Add/1
  Rate Transition1/1 -> Delay5/1, Multiply2/2
  Delay/1 -> Rate Transition/1
  Delay2/1 -> Add1/2
  Delay3/1 -> Add/2
  Delay7/1 -> Add3/2
  Add2/1 -> Delay2/1
  Add1/1 -> Delay3/1
  Rate Transition2/1 -> Delay6/1, Multiply3/2
  Delay1/1 -> Rate Transition1/1
  LoD_10/1 -> Multiply5/1
  Rate Transition/1 -> Delay1/1, Multiply1/2
  LoD_4/1 -> Multiply2/1
  Delay5/1 -> Rate Transition2/1
  LoD_0/1 -> Multiply/1
  LoD_2/1 -> Multiply1/1
  Delay8/1 -> Rate Transition4/1
  Rate Transition4/1 -> Multiply5/2
  Multiply4/1 -> Add4/1
  Delay4/1 -> Add2/2
  Delay9/1 -> Add4/2
  Multiply5/1 -> Delay9/1
  Delay6/1 -> Rate Transition3/1
  Add4/1 -> Delay7/1
  LoD_8/1 -> Multiply4/1
  LoD_6/1 -> Multiply3/1
  Multiply1/1 -> Add1/1

== system db6_4_Level_double/4th_Level_Decomp/LoD_Odd ==
  In_LoD_o : Inport  OutDataTypeStr=double  SampleTime=1/44100
  Add{,1..4} (5 alike) : Sum  AccumDataTypeStr=double  OutDataTypeStr=double
  Delay{,1..9} (10 alike) : Delay  DelayLength=1  SampleTime=1/44100
  LoD_1 : Constant  Value=0.004777258  OutDataTypeStr=double  SampleTime=1/44100
  LoD_11 : Constant  Value=0.111540743  OutDataTypeStr=double  SampleTime=1/44100
  LoD_3 : Constant  Value=-0.031582039  OutDataTypeStr=double  SampleTime=1/44100
  LoD_5 : Constant  Value=0.097501606  OutDataTypeStr=double  SampleTime=1/44100
  LoD_7 : Constant  Value=-0.226264694  OutDataTypeStr=double  SampleTime=1/44100
  LoD_9 : Constant  Value=0.751133908  OutDataTypeStr=double  SampleTime=1/44100
  Multiply{,1..5} (6 alike) : Product  OutDataTypeStr=double
  Rate Transition{,1..4} (5 alike) : RateTransition  OutPortSampleTime=1/44100
  Out_LoD_o : Outport  OutDataTypeStr=double  SampleTime=1/44100  VectorParamsAs1DForOutWhenUnconnected=off
  wires:
  LoD_1/1 -> Multiply/1
  Delay/1 -> Rate Transition/1
  Multiply4/1 -> Add4/1
  Delay2/1 -> Add1/2
  Rate Transition2/1 -> Delay6/1, Multiply3/2
  LoD_7/1 -> Multiply3/1
  Delay7/1 -> Add3/2
  Add2/1 -> Delay2/1
  Add1/1 -> Delay3/1
  Delay3/1 -> Add/2
  Multiply5/1 -> Delay9/1
  Rate Transition4/1 -> Multiply5/2
  Delay8/1 -> Rate Transition4/1
  Delay9/1 -> Add4/2
  Delay5/1 -> Rate Transition2/1
  Add4/1 -> Delay7/1
  Rate Transition3/1 -> Delay8/1, Multiply4/2
  LoD_9/1 -> Multiply4/1
  LoD_5/1 -> Multiply2/1
  Rate Transition/1 -> Delay1/1, Multiply1/2
  LoD_3/1 -> Multiply1/1
  Multiply3/1 -> Add3/1
  Delay1/1 -> Rate Transition1/1
  Add3/1 -> Delay4/1
  Multiply/1 -> Add/1
  Multiply1/1 -> Add1/1
  In_LoD_o/1 -> Delay/1, Multiply/2
  Delay6/1 -> Rate Transition3/1
  Delay4/1 -> Add2/2
  Add/1 -> Out_LoD_o/1
  LoD_11/1 -> Multiply5/1
  Multiply2/1 -> Add2/1
  Rate Transition1/1 -> Delay5/1, Multiply2/2

== system db6_4_Level_double/4th_Level_Recon/HiR_Even ==
  In_HiR_e : Inport  OutDataTypeStr=double  SampleTime=1/44100
  Add{,1..4} (5 alike) : Sum  AccumDataTypeStr=double  OutDataTypeStr=double
  Delay{,1..9} (10 alike) : Delay  DelayLength=1  SampleTime=1/44100
  HiR_0 : Constant  Value=-0.001077301  OutDataTypeStr=double  SampleTime=1/44100
  HiR_10 : Constant  Value=0.49462389  OutDataTypeStr=double  SampleTime=1/44100
  HiR_2 : Constant  Value=0.000553842  OutDataTypeStr=double  SampleTime=1/44100
  HiR_4 : Constant  Value=0.027522866  OutDataTypeStr=double  SampleTime=1/44100
  HiR_6 : Constant  Value=-0.129766868  OutDataTypeStr=double  SampleTime=1/44100
  HiR_8 : Constant  Value=0.315250352  OutDataTypeStr=double  SampleTime=1/44100
  Multiply{,1..5} (6 alike) : Product  OutDataTypeStr=double
  Rate Transition{,1..4} (5 alike) : RateTransition  OutPortSampleTime=1/44100
  Out_HiR_e : Outport  OutDataTypeStr=double  SampleTime=1/44100  VectorParamsAs1DForOutWhenUnconnected=off
  wires:
  Delay3/1 -> Add/2
  In_HiR_e/1 -> Delay/1, Multiply/2
  HiR_4/1 -> Multiply2/1
  Multiply/1 -> Add/1
  Add1/1 -> Delay3/1
  Multiply1/1 -> Add1/1
  Delay2/1 -> Add1/2
  Add/1 -> Out_HiR_e/1
  HiR_0/1 -> Multiply/1
  HiR_2/1 -> Multiply1/1
  Delay1/1 -> Rate Transition1/1
  Rate Transition/1 -> Delay1/1, Multiply1/2
  Rate Transition1/1 -> Delay4/1, Multiply2/2
  Delay/1 -> Rate Transition/1
  Delay4/1 -> Rate Transition2/1
  HiR_6/1 -> Multiply3/1
  Multiply2/1 -> Add2/1
  Add2/1 -> Delay2/1
  Delay5/1 -> Add2/2
  HiR_8/1 -> Multiply4/1
  Rate Transition2/1 -> Delay6/1, Multiply3/2
  Delay6/1 -> Rate Transition3/1
  Add3/1 -> Delay5/1
  Multiply3/1 -> Add3/1
  Delay7/1 -> Add3/2
  HiR_10/1 -> Multiply5/1
  Rate Transition3/1 -> Delay8/1, Multiply4/2
  Rate Transition4/1 -> Multiply5/2
  Delay8/1 -> Rate Transition4/1
  Multiply5/1 -> Delay9/1
  Add4/1 -> Delay7/1
  Multiply4/1 -> Add4/1
  Delay9/1 -> Add4/2

== system db6_4_Level_double/4th_Level_Recon/HiR_Odd ==
  In_HiR_o : Inport  OutDataTypeStr=double  SampleTime=1/44100
  Add{,1..4} (5 alike) : Sum  AccumDataTypeStr=double  OutDataTypeStr=double
  Delay{,1..9} (10 alike) : Delay  DelayLength=1  SampleTime=1/44100
  HiR_1 : Constant  Value=-0.004777258  OutDataTypeStr=double  SampleTime=1/44100
  HiR_11 : Constant  Value=-0.111540743  OutDataTypeStr=double  SampleTime=1/44100
  HiR_3 : Constant  Value=0.031582039  OutDataTypeStr=double  SampleTime=1/44100
  HiR_5 : Constant  Value=-0.097501606  OutDataTypeStr=double  SampleTime=1/44100
  HiR_7 : Constant  Value=0.226264694  OutDataTypeStr=double  SampleTime=1/44100
  HiR_9 : Constant  Value=-0.751133908  OutDataTypeStr=double  SampleTime=1/44100
  Multiply{,1..5} (6 alike) : Product  OutDataTypeStr=double
  Rate Transition{,1..4} (5 alike) : RateTransition  OutPortSampleTime=1/44100
  Out_HiR_o : Outport  OutDataTypeStr=double  SampleTime=1/44100  VectorParamsAs1DForOutWhenUnconnected=off
  wires:
  HiR_7/1 -> Multiply3/1
  HiR_3/1 -> Multiply1/1
  Delay2/1 -> Add1/2
  Delay/1 -> Rate Transition/1
  Delay5/1 -> Add2/2
  HiR_5/1 -> Multiply2/1
  Delay4/1 -> Rate Transition2/1
  Delay3/1 -> Add/2
  Add2/1 -> Delay2/1
  Multiply/1 -> Add/1
  Multiply1/1 -> Add1/1
  Rate Transition2/1 -> Delay6/1, Multiply3/2
  HiR_1/1 -> Multiply/1
  Multiply5/1 -> Delay9/1
  Delay1/1 -> Rate Transition1/1
  Delay8/1 -> Rate Transition4/1
  Add1/1 -> Delay3/1
  Add4/1 -> Delay7/1
  Delay9/1 -> Add4/2
  Rate Transition1/1 -> Delay4/1, Multiply2/2
  Add3/1 -> Delay5/1
  Delay6/1 -> Rate Transition3/1
  Rate Transition/1 -> Delay1/1, Multiply1/2
  HiR_9/1 -> Multiply4/1
  Multiply4/1 -> Add4/1
  Delay7/1 -> Add3/2
  Multiply3/1 -> Add3/1
  Multiply2/1 -> Add2/1
  HiR_11/1 -> Multiply5/1
  Rate Transition3/1 -> Delay8/1, Multiply4/2
  Add/1 -> Out_HiR_o/1
  In_HiR_o/1 -> Delay/1, Multiply/2
  Rate Transition4/1 -> Multiply5/2

== system db6_4_Level_double/4th_Level_Recon/LoR_Even ==
  In_LoR_e : Inport  OutDataTypeStr=double  SampleTime=1/44100
  Add{,1..4} (5 alike) : Sum  AccumDataTypeStr=double  OutDataTypeStr=double
  Delay{,1..9} (10 alike) : Delay  DelayLength=1  SampleTime=1/44100
  LoR_0 : Constant  Value=0.111540743  OutDataTypeStr=double  SampleTime=1/44100
  LoR_10 : Constant  Value=0.004777258  OutDataTypeStr=double  SampleTime=1/44100
  LoR_2 : Constant  Value=0.751133908  OutDataTypeStr=double  SampleTime=1/44100
  LoR_4 : Constant  Value=-0.226264694  OutDataTypeStr=double  SampleTime=1/44100
  LoR_6 : Constant  Value=0.097501606  OutDataTypeStr=double  SampleTime=1/44100
  LoR_8 : Constant  Value=-0.031582039  OutDataTypeStr=double  SampleTime=1/44100
  Multiply{,1..5} (6 alike) : Product  OutDataTypeStr=double
  Rate Transition{,1..4} (5 alike) : RateTransition  OutPortSampleTime=1/44100
  Out_LoR_e : Outport  OutDataTypeStr=double  SampleTime=1/44100  VectorParamsAs1DForOutWhenUnconnected=off
  wires:
  Multiply5/1 -> Delay9/1
  LoR_6/1 -> Multiply3/1
  Rate Transition2/1 -> Delay6/1, Multiply3/2
  Multiply1/1 -> Add1/1
  Multiply/1 -> Add/1
  LoR_8/1 -> Multiply4/1
  Rate Transition3/1 -> Delay8/1, Multiply4/2
  Add2/1 -> Delay2/1
  Delay5/1 -> Add2/2
  Multiply2/1 -> Add2/1
  Delay3/1 -> Add/2
  Delay4/1 -> Rate Transition2/1
  Delay2/1 -> Add1/2
  Delay/1 -> Rate Transition/1
  In_LoR_e/1 -> Delay/1, Multiply/2
  Rate Transition/1 -> Delay1/1, Multiply1/2
  Add1/1 -> Delay3/1
  Add3/1 -> Delay5/1
  Delay8/1 -> Rate Transition4/1
  Delay1/1 -> Rate Transition1/1
  Delay6/1 -> Rate Transition3/1
  Rate Transition1/1 -> Delay4/1, Multiply2/2
  Delay9/1 -> Add4/2
  LoR_4/1 -> Multiply2/1
  Add4/1 -> Delay7/1
  LoR_0/1 -> Multiply/1
  Rate Transition4/1 -> Multiply5/2
  Multiply3/1 -> Add3/1
  Multiply4/1 -> Add4/1
  LoR_2/1 -> Multiply1/1
  Delay7/1 -> Add3/2
  LoR_10/1 -> Multiply5/1
  Add/1 -> Out_LoR_e/1

== system db6_4_Level_double/4th_Level_Recon/LoR_Odd ==
  In_LoR_o : Inport  OutDataTypeStr=double  SampleTime=1/44100
  Add{,1..4} (5 alike) : Sum  AccumDataTypeStr=double  OutDataTypeStr=double
  Delay{,1..9} (10 alike) : Delay  DelayLength=1  SampleTime=1/44100
  LoR_1 : Constant  Value=0.49462389  OutDataTypeStr=double  SampleTime=1/44100
  LoR_11 : Constant  Value=-0.001077301  OutDataTypeStr=double  SampleTime=1/44100
  LoR_3 : Constant  Value=0.315250352  OutDataTypeStr=double  SampleTime=1/44100
  LoR_5 : Constant  Value=-0.129766868  OutDataTypeStr=double  SampleTime=1/44100
  LoR_7 : Constant  Value=0.027522866  OutDataTypeStr=double  SampleTime=1/44100
  LoR_9 : Constant  Value=0.000553842  OutDataTypeStr=double  SampleTime=1/44100
  Multiply{,1..5} (6 alike) : Product  OutDataTypeStr=double
  Rate Transition{,1..4} (5 alike) : RateTransition  OutPortSampleTime=1/44100
  Out_LoR_o : Outport  OutDataTypeStr=double  SampleTime=1/44100  VectorParamsAs1DForOutWhenUnconnected=off
  wires:
  Rate Transition2/1 -> Delay6/1, Multiply3/2
  Delay3/1 -> Add/2
  Add2/1 -> Delay2/1
  Delay4/1 -> Rate Transition2/1
  Delay/1 -> Rate Transition/1
  Delay5/1 -> Add2/2
  Delay2/1 -> Add1/2
  LoR_5/1 -> Multiply2/1
  LoR_7/1 -> Multiply3/1
  LoR_1/1 -> Multiply/1
  Multiply5/1 -> Delay9/1
  Multiply4/1 -> Add4/1
  LoR_11/1 -> Multiply5/1
  Rate Transition/1 -> Delay1/1, Multiply1/2
  Multiply/1 -> Add/1
  Delay6/1 -> Rate Transition3/1
  Add3/1 -> Delay5/1
  Rate Transition1/1 -> Delay4/1, Multiply2/2
  Add4/1 -> Delay7/1
  Delay9/1 -> Add4/2
  Add1/1 -> Delay3/1
  Delay8/1 -> Rate Transition4/1
  In_LoR_o/1 -> Delay/1, Multiply/2
  Add/1 -> Out_LoR_o/1
  Rate Transition3/1 -> Delay8/1, Multiply4/2
  Multiply1/1 -> Add1/1
  Rate Transition4/1 -> Multiply5/2
  LoR_9/1 -> Multiply4/1
  Delay1/1 -> Rate Transition1/1
  Delay7/1 -> Add3/2
  LoR_3/1 -> Multiply1/1
  Multiply3/1 -> Add3/1
  Multiply2/1 -> Add2/1

== system db6_4_Level_double/Threshold_Estimator/Absolute_Value1 ==
  Signal_w4 : Inport  OutDataTypeStr=double  SampleTime=1/44100
  Absolute_Switch : Switch  Threshold=1  OutDataTypeStr=double
  Constant295 : Constant  Value=0  OutDataTypeStr=double  SampleTime=1/44100
  Gain2 : Gain  Gain=-1  ParamDataTypeStr=double  OutDataTypeStr=double
  Relational Operator2 : RelationalOperator  Operator=<  OutDataTypeStr=boolean  RndMeth=Simplest
  Out_Abs : Outport  OutDataTypeStr=double  SampleTime=1/44100  VectorParamsAs1DForOutWhenUnconnected=off
  wires:
  Absolute_Switch/1 -> Out_Abs/1
  Relational Operator2/1 -> Absolute_Switch/2
  Gain2/1 -> Absolute_Switch/1
  Signal_w4/1 -> Absolute_Switch/3, Relational Operator2/1, Gain2/1
  Constant295/1 -> Relational Operator2/2

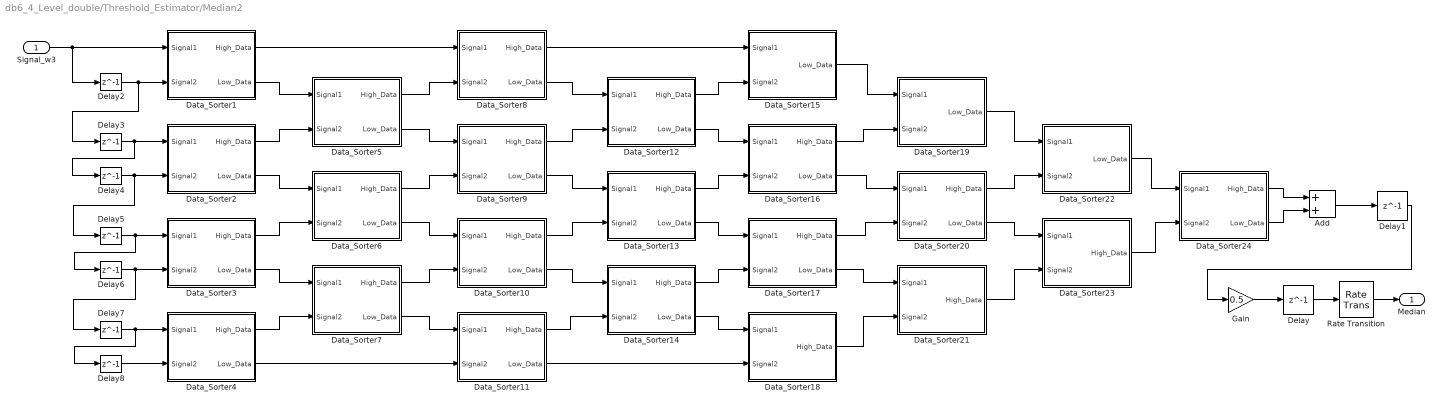
== system db6_4_Level_double/Threshold_Estimator/Median2 ==
  Signal_w3 : Inport  OutDataTypeStr=double  SampleTime=1/44100
  Add : Sum  AccumDataTypeStr=double  OutDataTypeStr=double  LockScale=on
  Data_Sorter1 : Subsystem
  Data_Sorter10 : Subsystem
  Data_Sorter11 : Subsystem
  Data_Sorter12 : Subsystem
  Data_Sorter13 : Subsystem
  Data_Sorter14 : Subsystem
  Data_Sorter15 : Subsystem
  Data_Sorter16 : Subsystem
  Data_Sorter17 : Subsystem
  Data_Sorter18 : Subsystem
  Data_Sorter19 : Subsystem
  Data_Sorter2 : Subsystem
  Data_Sorter20 : Subsystem
  Data_Sorter21 : Subsystem
  Data_Sorter22 : Subsystem
  Data_Sorter23 : Subsystem
  Data_Sorter24 : Subsystem
  Data_Sorter3 : Subsystem
  Data_Sorter4 : Subsystem
  Data_Sorter5 : Subsystem
  Data_Sorter6 : Subsystem
  Data_Sorter7 : Subsystem
  Data_Sorter8 : Subsystem
  Data_Sorter9 : Subsystem
  Delay{,1..8} (9 alike) : Delay  DelayLength=1  SampleTime=1/44100
  Gain : Gain  Gain=0.5  ParamDataTypeStr=double  OutDataTypeStr=double
  Rate Transition : RateTransition  OutPortSampleTime=1/44100
  Median : Outport  OutDataTypeStr=double  SampleTime=1/44100  VectorParamsAs1DForOutWhenUnconnected=off
  wires:
  Data_Sorter4/1(High_Data) -> Data_Sorter7/2(Signal2)
  Delay3/1 -> Data_Sorter2/1(Signal1), Delay4/1
  Signal_w3/1 -> Data_Sorter1/1(Signal1), Delay2/1
  Data_Sorter10/1(High_Data) -> Data_Sorter13/2(Signal2)
  Data_Sorter23/1(High_Data) -> Data_Sorter24/2(Signal2)
  Data_Sorter12/2(Low_Data) -> Data_Sorter16/1(Signal1)
  Delay2/1 -> Delay3/1, Data_Sorter1/2(Signal2)
  Data_Sorter5/1(High_Data) -> Data_Sorter8/2(Signal2)
  Delay/1 -> Rate Transition/1
  Data_Sorter15/1(Low_Data) -> Data_Sorter19/1(Signal1)
  Add/1 -> Delay1/1
  Data_Sorter7/2(Low_Data) -> Data_Sorter11/1(Signal1)
  Data_Sorter24/1(High_Data) -> Add/1
  Data_Sorter1/2(Low_Data) -> Data_Sorter5/1(Signal1)
  Data_Sorter3/1(High_Data) -> Data_Sorter6/2(Signal2)
  Data_Sorter22/1(Low_Data) -> Data_Sorter24/1(Signal1)
  Data_Sorter2/1(High_Data) -> Data_Sorter5/2(Signal2)
  Data_Sorter10/2(Low_Data) -> Data_Sorter14/1(Signal1)
  Delay1/1 -> Gain/1
  Data_Sorter17/2(Low_Data) -> Data_Sorter21/1(Signal1)
  Data_Sorter21/1(High_Data) -> Data_Sorter23/2(Signal2)
  Data_Sorter7/1(High_Data) -> Data_Sorter10/2(Signal2)
  Delay4/1 -> Data_Sorter2/2(Signal2), Delay5/1
  Data_Sorter16/1(High_Data) -> Data_Sorter19/2(Signal2)
  Data_Sorter20/1(High_Data) -> Data_Sorter22/2(Signal2)
  Data_Sorter16/2(Low_Data) -> Data_Sorter20/1(Signal1)
  Data_Sorter3/2(Low_Data) -> Data_Sorter7/1(Signal1)
  Data_Sorter2/2(Low_Data) -> Data_Sorter6/1(Signal1)
  Data_Sorter6/2(Low_Data) -> Data_Sorter10/1(Signal1)
  Data_Sorter19/1(Low_Data) -> Data_Sorter22/1(Signal1)
  Data_Sorter12/1(High_Data) -> Data_Sorter15/2(Signal2)
  Data_Sorter5/2(Low_Data) -> Data_Sorter9/1(Signal1)
  Data_Sorter24/2(Low_Data) -> Add/2
  Data_Sorter17/1(High_Data) -> Data_Sorter20/2(Signal2)
  Data_Sorter13/1(High_Data) -> Data_Sorter16/2(Signal2)
  Data_Sorter11/1(High_Data) -> Data_Sorter14/2(Signal2)
  Delay8/1 -> Data_Sorter4/2(Signal2)
  Data_Sorter8/2(Low_Data) -> Data_Sorter12/1(Signal1)
  Delay6/1 -> Data_Sorter3/2(Signal2), Delay7/1
  Data_Sorter9/2(Low_Data) -> Data_Sorter13/1(Signal1)
  Data_Sorter4/2(Low_Data) -> Data_Sorter11/2(Signal2)
  Data_Sorter9/1(High_Data) -> Data_Sorter12/2(Signal2)
  Data_Sorter14/2(Low_Data) -> Data_Sorter18/1(Signal1)
  Delay5/1 -> Data_Sorter3/1(Signal1), Delay6/1
  Delay7/1 -> Data_Sorter4/1(Signal1), Delay8/1
  Data_Sorter1/1(High_Data) -> Data_Sorter8/1(Signal1)
  Data_Sorter8/1(High_Data) -> Data_Sorter15/1(Signal1)
  Data_Sorter14/1(High_Data) -> Data_Sorter17/2(Signal2)
  Data_Sorter6/1(High_Data) -> Data_Sorter9/2(Signal2)
  Data_Sorter20/2(Low_Data) -> Data_Sorter23/1(Signal1)
  Data_Sorter11/2(Low_Data) -> Data_Sorter18/2(Signal2)
  Data_Sorter13/2(Low_Data) -> Data_Sorter17/1(Signal1)
  Gain/1 -> Delay/1
  Data_Sorter18/1(High_Data) -> Data_Sorter21/2(Signal2)
  Rate Transition/1 -> Median/1

== system db6_4_Level_double/Threshold_Estimator/Median2/Data_Sorter1 ==
  Signal1 : Inport  OutDataTypeStr=double  SampleTime=1/44100
  Signal2 : Inport  Port=2  OutDataTypeStr=double  SampleTime=1/44100
  Data_Sorter_Switch : Switch  OutDataTypeStr=double
  Data_Sorter_Switch1 : Switch  Threshold=1  OutDataTypeStr=double
  Delay1 : Delay  DelayLength=1  SampleTime=1/44100
  Delay2 : Delay  DelayLength=1  SampleTime=1/44100
  Relational Operator2 : RelationalOperator  Operator=<  OutDataTypeStr=boolean  RndMeth=Simplest
  High_Data : Outport  OutDataTypeStr=double  SampleTime=1/44100  VectorParamsAs1DForOutWhenUnconnected=off
  Low_Data : Outport  Port=2  OutDataTypeStr=double  SampleTime=1/44100  VectorParamsAs1DForOutWhenUnconnected=off
  wires:
  Signal1/1 -> Data_Sorter_Switch/3, Data_Sorter_Switch/1, Relational Operator2/1
  Relational Operator2/1 -> Data_Sorter_Switch1/2, Data_Sorter_Switch/2
  Signal2/1 -> Data_Sorter_Switch1/1, Data_Sorter_Switch1/3, Relational Operator2/2
  Data_Sorter_Switch1/1 -> Delay2/1
  Delay2/1 -> Low_Data/1
  Data_Sorter_Switch/1 -> Delay1/1
  Delay1/1 -> High_Data/1

== system db6_4_Level_double/Threshold_Estimator/Median2/Data_Sorter10 ==
  Signal1 : Inport  OutDataTypeStr=double  SampleTime=1/44100
  Signal2 : Inport  Port=2  OutDataTypeStr=double  SampleTime=1/44100
  Data_Sorter_Switch : Switch  OutDataTypeStr=double
  Data_Sorter_Switch1 : Switch  Threshold=1  OutDataTypeStr=double
  Delay1 : Delay  DelayLength=1  SampleTime=1/44100
  Delay2 : Delay  DelayLength=1  SampleTime=1/44100
  Relational Operator2 : RelationalOperator  Operator=<  OutDataTypeStr=boolean  RndMeth=Simplest
  High_Data : Outport  OutDataTypeStr=double  SampleTime=1/44100  VectorParamsAs1DForOutWhenUnconnected=off
  Low_Data : Outport  Port=2  OutDataTypeStr=double  SampleTime=1/44100  VectorParamsAs1DForOutWhenUnconnected=off
  wires:
  Signal1/1 -> Data_Sorter_Switch/3, Data_Sorter_Switch/1, Relational Operator2/1
  Relational Operator2/1 -> Data_Sorter_Switch1/2, Data_Sorter_Switch/2
  Signal2/1 -> Data_Sorter_Switch1/1, Data_Sorter_Switch1/3, Relational Operator2/2
  Data_Sorter_Switch1/1 -> Delay2/1
  Delay2/1 -> Low_Data/1
  Data_Sorter_Switch/1 -> Delay1/1
  Delay1/1 -> High_Data/1
